simulink model "motorExpIdent"  (R2022a)
settings: Solver=VariableStepAuto  StartTime=0.0  StopTime=10.0  RelTol=1e-3
values from neighbouring files (symbols this model uses):
  K = 114.4795944    [MotorExpScriptIdent.m]    (also in motorSimScript.m = 8; motorSimScriptIdent.m = 10)
  sigma = 0.1147802808    [MotorExpScriptIdent.m]    (also in motorSimScript.m = 0.2; motorSimScriptIdent.m = 0.2)
settings Model: Creator=coffe  LastModifiedBy=coffe
settings SolverCC: AlgebraicLoopSolver=TrustRegion
settings DebuggingCC: UnconnectedInputMsg=warning  UnconnectedOutputMsg=warning  UnconnectedLineMsg=warning  SFMachineParentedDataDiag=warning

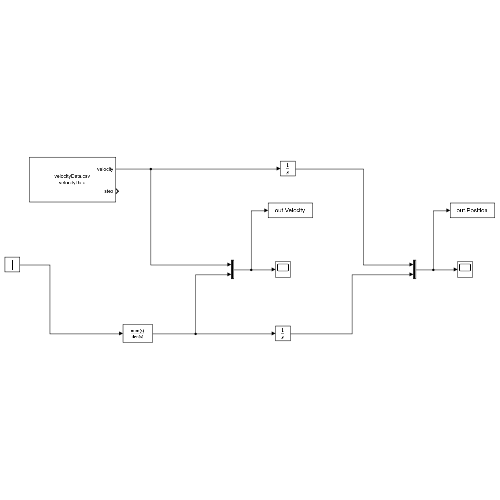
[thumbnail: Simulink's stored preview of the top-level diagram]
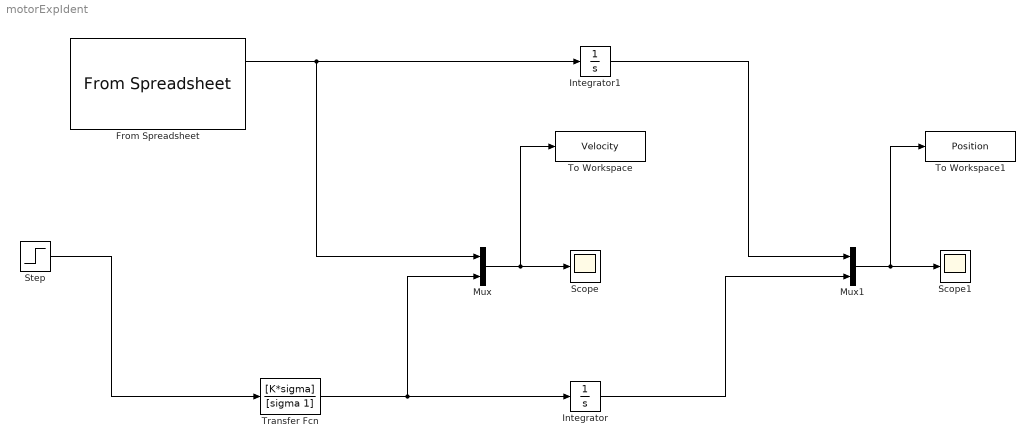
== system motorExpIdent ==
  From Spreadsheet : FromSpreadsheet  FileName=velocityData.csv  SheetName=velocityData  OutDataTypeStr=double
  Integrator : Integrator
  Integrator1 : Integrator
  Mux : Mux  Inputs=2
  Mux1 : Mux  Inputs=2
  Scope : Scope
  Scope1 : Scope
  Step : Step  SampleTime=0
  To Workspace : ToWorkspace  VariableName=Velocity  SaveFormat=Timeseries  SampleTime=-1
  To Workspace1 : ToWorkspace  VariableName=Position  SaveFormat=Timeseries  SampleTime=-1
  Transfer Fcn : TransferFcn  Numerator=[K*sigma]  Denominator=[sigma 1]
  wires:
  Mux/1 -> Scope/1, To Workspace/1
  Mux1/1 -> Scope1/1, To Workspace1/1
  Step/1 -> Transfer Fcn/1
  From Spreadsheet/1 -> Mux/1, Integrator1/1
  Integrator/1 -> Mux1/2
  Transfer Fcn/1 -> Mux/2, Integrator/1
  Integrator1/1 -> Mux1/1
